simulink model "Exemplo_de_integrador"  (R2022a)
settings: Solver=VariableStepAuto  StartTime=0.0  StopTime=50  RelTol=1e-3
settings Model: Creator=souza  LastModifiedBy=souza

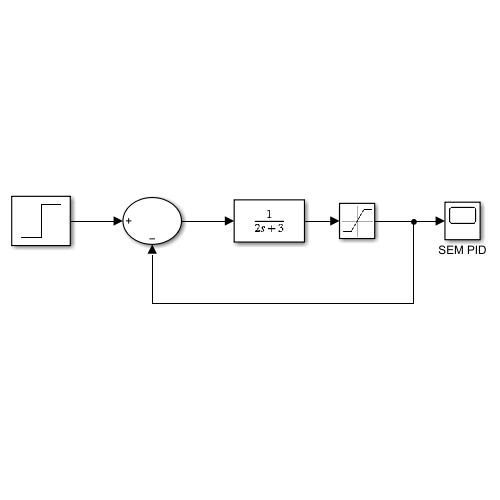
[thumbnail: Simulink's stored preview of the top-level diagram]
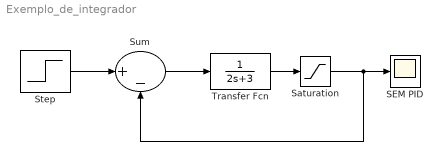
== system Exemplo_de_integrador ==
  SEM PID : Scope
  Saturation : Saturate  UpperLimit=5  LowerLimit=0
  Step : Step  Time=0  After=3  SampleTime=0
  Sum : Sum  Inputs=|+-
  Transfer Fcn : TransferFcn  Denominator=[2 3]  ParameterTunability=Optimized
  wires:
  Step/1 -> Sum/1
  Sum/1 -> Transfer Fcn/1
  Transfer Fcn/1 -> Saturation/1
  Saturation/1 -> SEM PID/1, Sum/2
